simulink model "huzeyfe_ivot_462"  (R2018a)
settings: Solver=VariableStepAuto  StartTime=0.0  StopTime=10.0  RelTol=1e-3
libraries: powerlib x21, simulink x3, powerlib_meascontrol x1
settings Model: Creator=Gulten  LastModifiedBy=Gulten

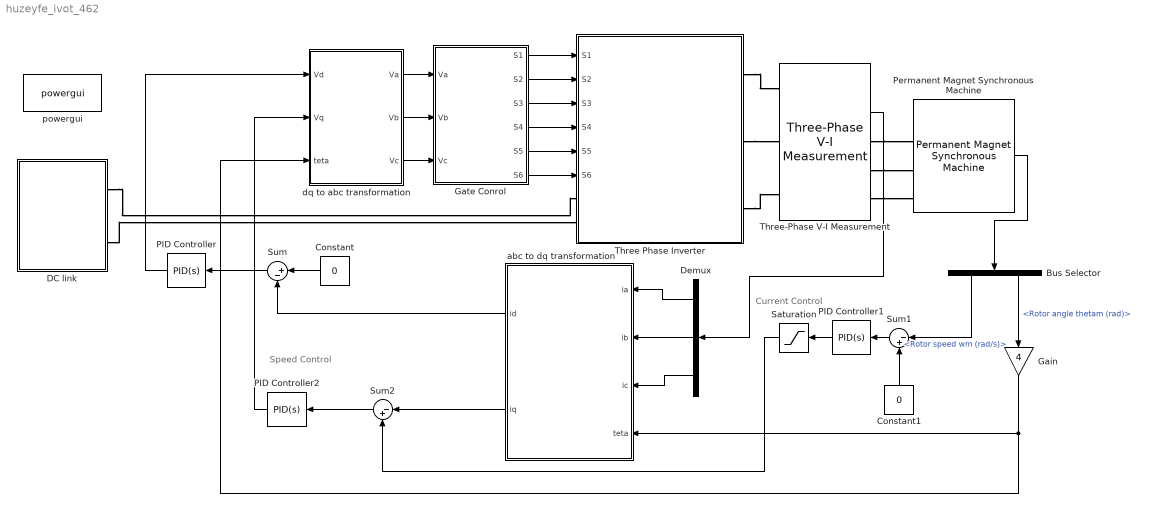
== system huzeyfe_ivot_462 ==
  note: Speed Control
  note: Current Control
  Bus Selector : BusSelector  OutputSignals=Rotor speed wm (rad/s),Rotor angle thetam (rad)
  Constant : Constant  Value=0
  Constant1 : Constant  Value=0
  DC link : Subsystem
  Demux : Demux  Outputs=3
  Gain : Gain  Gain=4
  Gate Conrol : Subsystem
  PID Controller : simulink/Continuous/PID Controller  Controller=PID  TimeDomain=Continuous-time  SampleTime=-1  IntegratorMethod=Forward Euler  FilterMethod=Forward Euler  Form=Parallel  UseFilter=on  ControllerParametersSource=internal  P=1  I=1  D=0  N=100  InitialConditionSource=internal  InitialConditionForIntegrator=0  InitialConditionForFilter=0  ExternalReset=none  LimitOutput=off  UpperSaturationLimit=inf  LowerSaturationLimit=-inf  LinearizeAsGain=on  AntiWindupMode=none  Kb=1  TrackingMode=off  Kt=1  PParamMin=[]  PParamMax=[]  IParamMin=[]  IParamMax=[]  DParamMin=[]  DParamMax=[]  NParamMin=[]  NParamMax=[]  KbParamMin=[]  KbParamMax=[]  KtParamMin=[]  KtParamMax=[]  POutMin=[]  POutMax=[]  IOutMin=[]  IOutMax=[]  DOutMin=[]  DOutMax=[]  NOutMin=[]  NOutMax=[]  KbOutMin=[]  KbOutMax=[]  KtOutMin=[]  KtOutMax=[]  IntegratorOutMin=[]  IntegratorOutMax=[]  FilterOutMin=[]  FilterOutMax=[]  SumOutMin=[]  SumOutMax=[]  SumI1OutMin=[]  SumI1OutMax=[]  SumI2OutMin=[]  SumI2OutMax=[]  SumI3OutMin=[]  SumI3OutMax=[]  SumDOutMin=[]  SumDOutMax=[]  SaturationOutMin=[]  SaturationOutMax=[]  IntegratorContinuousStateAttributes=''  IntegratorStateMustResolveToSignalObject=off  IntegratorRTWStateStorageClass=Auto  FilterContinuousStateAttributes=''  FilterStateMustResolveToSignalObject=off  FilterRTWStateStorageClass=Auto  DifferentiatorICPrevScaledInput=0  DifferentiatorOutMin=[]  DifferentiatorOutMax=[]  FilterDiffOutCoefMin=[]  FilterDiffOutCoefMax=[]  SumDenOutMin=[]  SumDenOutMax=[]  SumNumOutMin=[]  SumNumOutMax=[]  ReciprocalOutMin=[]  ReciprocalOutMax=[]  DivideOutMin=[]  DivideOutMax=[]  TunerSelectOption=Transfer Function Based (PID Tuner App)
  PID Controller1 : simulink/Continuous/PID Controller  Controller=PID  TimeDomain=Continuous-time  SampleTime=-1  IntegratorMethod=Forward Euler  FilterMethod=Forward Euler  Form=Parallel  UseFilter=on  ControllerParametersSource=internal  P=1  I=1  D=0  N=100  InitialConditionSource=internal  InitialConditionForIntegrator=0  InitialConditionForFilter=0  ExternalReset=none  LimitOutput=off  UpperSaturationLimit=inf  LowerSaturationLimit=-inf  LinearizeAsGain=on  AntiWindupMode=none  Kb=1  TrackingMode=off  Kt=1  PParamMin=[]  PParamMax=[]  IParamMin=[]  IParamMax=[]  DParamMin=[]  DParamMax=[]  NParamMin=[]  NParamMax=[]  KbParamMin=[]  KbParamMax=[]  KtParamMin=[]  KtParamMax=[]  POutMin=[]  POutMax=[]  IOutMin=[]  IOutMax=[]  DOutMin=[]  DOutMax=[]  NOutMin=[]  NOutMax=[]  KbOutMin=[]  KbOutMax=[]  KtOutMin=[]  KtOutMax=[]  IntegratorOutMin=[]  IntegratorOutMax=[]  FilterOutMin=[]  FilterOutMax=[]  SumOutMin=[]  SumOutMax=[]  SumI1OutMin=[]  SumI1OutMax=[]  SumI2OutMin=[]  SumI2OutMax=[]  SumI3OutMin=[]  SumI3OutMax=[]  SumDOutMin=[]  SumDOutMax=[]  SaturationOutMin=[]  SaturationOutMax=[]  IntegratorContinuousStateAttributes=''  IntegratorStateMustResolveToSignalObject=off  IntegratorRTWStateStorageClass=Auto  FilterContinuousStateAttributes=''  FilterStateMustResolveToSignalObject=off  FilterRTWStateStorageClass=Auto  DifferentiatorICPrevScaledInput=0  DifferentiatorOutMin=[]  DifferentiatorOutMax=[]  FilterDiffOutCoefMin=[]  FilterDiffOutCoefMax=[]  SumDenOutMin=[]  SumDenOutMax=[]  SumNumOutMin=[]  SumNumOutMax=[]  ReciprocalOutMin=[]  ReciprocalOutMax=[]  DivideOutMin=[]  DivideOutMax=[]  TunerSelectOption=Transfer Function Based (PID Tuner App)
  PID Controller2 : simulink/Continuous/PID Controller  Controller=PID  TimeDomain=Continuous-time  SampleTime=-1  IntegratorMethod=Forward Euler  FilterMethod=Forward Euler  Form=Parallel  UseFilter=on  ControllerParametersSource=internal  P=1  I=1  D=0  N=100  InitialConditionSource=internal  InitialConditionForIntegrator=0  InitialConditionForFilter=0  ExternalReset=none  LimitOutput=off  UpperSaturationLimit=inf  LowerSaturationLimit=-inf  LinearizeAsGain=on  AntiWindupMode=none  Kb=1  TrackingMode=off  Kt=1  PParamMin=[]  PParamMax=[]  IParamMin=[]  IParamMax=[]  DParamMin=[]  DParamMax=[]  NParamMin=[]  NParamMax=[]  KbParamMin=[]  KbParamMax=[]  KtParamMin=[]  KtParamMax=[]  POutMin=[]  POutMax=[]  IOutMin=[]  IOutMax=[]  DOutMin=[]  DOutMax=[]  NOutMin=[]  NOutMax=[]  KbOutMin=[]  KbOutMax=[]  KtOutMin=[]  KtOutMax=[]  IntegratorOutMin=[]  IntegratorOutMax=[]  FilterOutMin=[]  FilterOutMax=[]  SumOutMin=[]  SumOutMax=[]  SumI1OutMin=[]  SumI1OutMax=[]  SumI2OutMin=[]  SumI2OutMax=[]  SumI3OutMin=[]  SumI3OutMax=[]  SumDOutMin=[]  SumDOutMax=[]  SaturationOutMin=[]  SaturationOutMax=[]  IntegratorContinuousStateAttributes=''  IntegratorStateMustResolveToSignalObject=off  IntegratorRTWStateStorageClass=Auto  FilterContinuousStateAttributes=''  FilterStateMustResolveToSignalObject=off  FilterRTWStateStorageClass=Auto  DifferentiatorICPrevScaledInput=0  DifferentiatorOutMin=[]  DifferentiatorOutMax=[]  FilterDiffOutCoefMin=[]  FilterDiffOutCoefMax=[]  SumDenOutMin=[]  SumDenOutMax=[]  SumNumOutMin=[]  SumNumOutMax=[]  ReciprocalOutMin=[]  ReciprocalOutMax=[]  DivideOutMin=[]  DivideOutMax=[]  TunerSelectOption=Transfer Function Based (PID Tuner App)
  Permanent Magnet Synchronous Machine : powerlib/Machines/Permanent Magnet Synchronous Machine  NbPhases=3  FluxDistribution=Sinusoidal  RotorType=Round  MechanicalLoad=Torque Tm  PresetModel=No  ShowDetailedParameters=on  MeasurementBus=off  Resistance=50e-3  Inductance=8.5e-3  dqInductances=[500e-6,500e-6]  La=500e-6  MachineConstant=Flux linkage established by magnets (V.s)  Flux=0.2  VoltageCst=145.1039  TorqueCst=1.2  Flat=120  Mechanical=[10 0 4 0]  PolePairs=4  InitialConditions=[266,0, 0,0]  InitialConditions5ph=[266 0 0 0 0 0]  TsPowergui=0  TsBlock=-1  RefAngle=90 degrees behind phase A axis (modified Park)
      settings: SourceProductName=Simscape Power Systems
  Saturation : Saturate  UpperLimit=250  LowerLimit=-250
  Sum : Sum  Inputs=|+-
  Sum1 : Sum  Inputs=|-+
  Sum2 : Sum  Inputs=|-+
  Three Phase Inverter : Subsystem
  Three-Phase V-I Measurement : powerlib/Measurements/Three-Phase V-I Measurement  VoltageMeasurement=phase-to-phase  SetLabelV=off  LabelV=Vabc  Vpu=off  VpuLL=off  CurrentMeasurement=yes  SetLabelI=off  LabelI=Iabc  Ipu=off  Pbase=100e6  Vbase=500e3  OutputType=Complex  PhasorSimulation=off  PSBequivalent=0
  abc to dq transformation : Subsystem
  dq to abc transformation : Subsystem
  powergui : powerlib/powergui  Priority=1  SimulationMode=Discrete  SampleTime=5e-7  frequency=60  Iterations=50  frequencyindice=0  Pbase=100e6  ErrMax=1e-4  UnitsV=kV  UnitsW=MW  buscounter=0  FunctionMessages=off  echomessages=off  EnableUseOfTLC=off  CurrentSourceSwitches=off  DisableSnubberDevices=off  DisableRonSwitches=off  DisableVfSwitches=off  DisplayEquations=off  SolverType=Tustin/Backward Euler (TBE)  Interpol=off  ExternalGateDelay=off  methode=off  Ts=100  x0status=blocks  SPID=on  SwTol=0  HookPort=off  RestoreLinks=warning  ResistiveCurrentMeasurement=off  Frange=[0:2:500]  Ylog=off  Xlog=on  ShowGrid=off  save=off  variable=ZData  structure=0  ZoomFFT=off  StartTime=0.0  cycles=1  DisplayStyle=1  fundamental=60  FreqAxis=off  MaxFrequency=1000  frequencyindicesteady=1  RmsSteady=1  display=off
  wires:
  Gate Conrol/1(S1) -> Three Phase Inverter/1(S1)
  Gate Conrol/2(S2) -> Three Phase Inverter/2(S2)
  Gate Conrol/3(S3) -> Three Phase Inverter/3(S3)
  Gate Conrol/4(S4) -> Three Phase Inverter/4(S4)
  Gate Conrol/5(S5) -> Three Phase Inverter/5(S5)
  Gate Conrol/6(S6) -> Three Phase Inverter/6(S6)
  dq to abc transformation/1(Va) -> Gate Conrol/1(Va)
  dq to abc transformation/2(Vb) -> Gate Conrol/2(Vb)
  dq to abc transformation/3(Vc) -> Gate Conrol/3(Vc)
  Three-Phase V-I Measurement/2 -> Demux/1
  Demux/1 -> abc to dq transformation/1(ia)
  Demux/2 -> abc to dq transformation/2(ib)
  Demux/3 -> abc to dq transformation/3(ic)
  Permanent Magnet Synchronous Machine/1 -> Bus Selector/1
  Bus Selector/2 -> Gain/1  "<Rotor angle thetam (rad)>"
  abc to dq transformation/1(id) -> Sum/2
  Constant/1 -> Sum/1
  Sum/1 -> PID Controller/1
  PID Controller/1 -> dq to abc transformation/1(Vd)
  Gain/1 -> dq to abc transformation/3("teta "), abc to dq transformation/4(teta)
  Bus Selector/1 -> Sum1/1  "<Rotor speed wm (rad/s)>"
  Constant1/1 -> Sum1/2
  Sum1/1 -> PID Controller1/1
  abc to dq transformation/2(iq) -> Sum2/1
  Sum2/1 -> PID Controller2/1
  PID Controller2/1 -> dq to abc transformation/2(Vq)
  PID Controller1/1 -> Saturation/1
  Saturation/1 -> Sum2/2
  connections:
  DC link/RConn1 -- Three Phase Inverter/LConn1
  DC link/RConn2 -- Three Phase Inverter/LConn2
  Three Phase Inverter/RConn1 -- Three-Phase V-I Measurement/LConn1
  Three Phase Inverter/RConn2 -- Three-Phase V-I Measurement/LConn2
  Three Phase Inverter/RConn3 -- Three-Phase V-I Measurement/LConn3
  Three-Phase V-I Measurement/RConn1 -- Permanent Magnet Synchronous Machine/LConn1
  Three-Phase V-I Measurement/RConn2 -- Permanent Magnet Synchronous Machine/LConn2
  Three-Phase V-I Measurement/RConn3 -- Permanent Magnet Synchronous Machine/LConn3

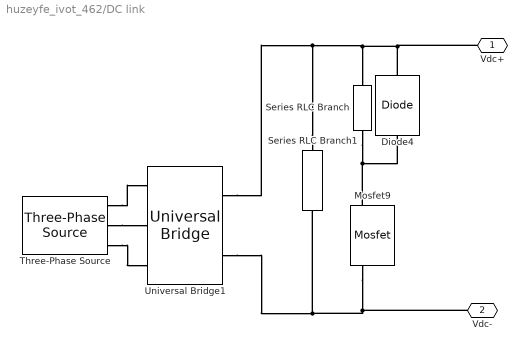
== system huzeyfe_ivot_462/DC link ==
  Diode4 : powerlib/Power Electronics/Diode  Ron=0.001  Lon=0  Vf=0  IC=0  UseSnubber=0  Rs=inf  Cs=inf  Measurements=off
  Mosfet9 : powerlib/Power Electronics/Mosfet  Ron=0.1  Lon=0  Rd=0.01  Vfd=0  IC=0  Rs=1e5  Cs=inf  Measurements=on
  Series RLC Branch : powerlib/Elements/Series RLC Branch  LConnTagsString=__new0  RConnTagsString=__new0  BranchType=R  Resistance=3  Inductance=1e-3  SetiL0=off  InitialCurrent=0  Capacitance=1e-6  Setx0=off  InitialVoltage=0  Measurements=None
  Series RLC Branch1 : powerlib/Elements/Series RLC Branch  LConnTagsString=__new0  RConnTagsString=__new0  BranchType=C  Resistance=1  Inductance=1e-3  SetiL0=off  InitialCurrent=0  Capacitance=1e-3  Setx0=off  InitialVoltage=0  Measurements=None
  Three-Phase Source : powerlib/Electrical Sources/Three-Phase Source  InternalConnection=Yg  VoltagePhases=off  Voltage=400  PhaseAngle=0  Voltage_phases=[25e3 25e3 25e3]/sqrt(3)  PhaseAngles_phases=[0 -120 +120]  Frequency=50  NonIdealSource=off  SpecifyImpedance=off  Resistance=0  Inductance=0  ShortCircuitLevel=100e6  BaseVoltage=25e3  XRratio=7  BusType=swing  Pref=10e3  Qref=0  Prefabc=[10e3, 10e3, 10e3]  Qrefabc=[0, 0, 0]  Qmin=-inf  Qmax=inf
  Universal Bridge1 : powerlib/Power Electronics/Universal Bridge  Arms=3  SnubberResistance=1e70  SnubberCapacitance=inf  Device=Diodes  Ron=1e-3  Lon=0  ForwardVoltages="[  0  0  ]"  ForwardVoltage=0  GTOparameters=[ 10e-6 , 20e-6 ]  IGBTparameters=[ 1e-6 , 2e-6 ]  Measurements=None  Measurements_2=None  converterType=Rectifier
  Vdc+ : PMIOPort  Side=Right
  Vdc- : PMIOPort  Port=2  Side=Right
  connections:
  Mosfet9/RConn1 -- Vdc-/RConn1 -- Universal Bridge1/RConn2 -- Series RLC Branch1/RConn1
  Series RLC Branch1/LConn1 -- Diode4/RConn1 -- Vdc+/RConn1 -- Series RLC Branch/LConn1 -- Universal Bridge1/RConn1
  Diode4/LConn1 -- Series RLC Branch/RConn1 -- Mosfet9/LConn1
  Three-Phase Source/RConn2 -- Universal Bridge1/LConn2
  Three-Phase Source/RConn3 -- Universal Bridge1/LConn3
  Three-Phase Source/RConn1 -- Universal Bridge1/LConn1

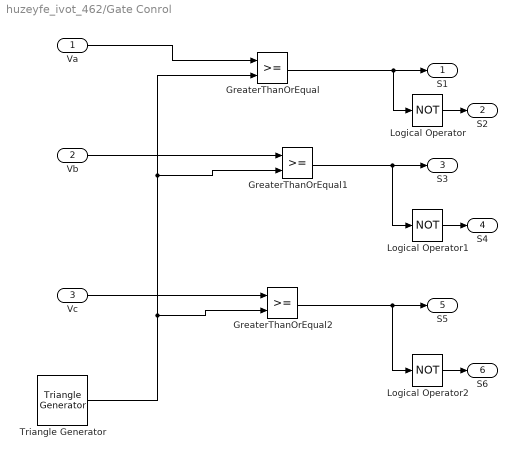
== system huzeyfe_ivot_462/Gate Conrol ==
  Va : Inport
  Vb : Inport  Port=2
  Vc : Inport  Port=3
  GreaterThanOrEqual : RelationalOperator  OutDataTypeStr=boolean  RndMeth=Simplest
  GreaterThanOrEqual1 : RelationalOperator  OutDataTypeStr=boolean  RndMeth=Simplest
  GreaterThanOrEqual2 : RelationalOperator  OutDataTypeStr=boolean  RndMeth=Simplest
  Logical Operator : Logic  Operator=NOT  AllPortsSameDT=off  OutDataTypeStr=boolean
  Logical Operator1 : Logic  Operator=NOT  AllPortsSameDT=off  OutDataTypeStr=boolean
  Logical Operator2 : Logic  Operator=NOT  AllPortsSameDT=off  OutDataTypeStr=boolean
  Triangle Generator : powerlib_meascontrol/Pulse & Signal Generators/Triangle Generator  Freq=5330  Phase=90  Ts=0
  S1 : Outport
  S2 : Outport  Port=2
  S3 : Outport  Port=3
  S4 : Outport  Port=4
  S5 : Outport  Port=5
  S6 : Outport  Port=6
  wires:
  Vc/1 -> GreaterThanOrEqual2/1
  Logical Operator2/1 -> S6/1
  Logical Operator1/1 -> S4/1
  Logical Operator/1 -> S2/1
  GreaterThanOrEqual1/1 -> S3/1, Logical Operator1/1
  GreaterThanOrEqual2/1 -> S5/1, Logical Operator2/1
  Va/1 -> GreaterThanOrEqual/1
  GreaterThanOrEqual/1 -> S1/1, Logical Operator/1
  Triangle Generator/1 -> GreaterThanOrEqual2/2, GreaterThanOrEqual/2, GreaterThanOrEqual1/2
  Vb/1 -> GreaterThanOrEqual1/1

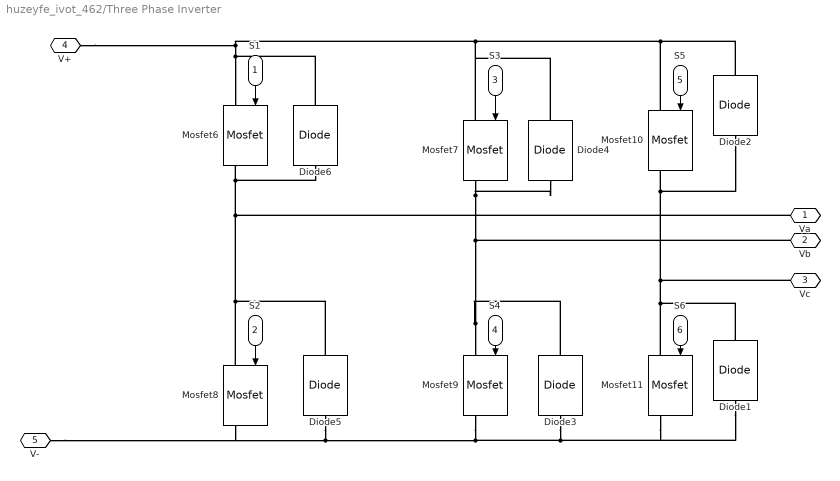
== system huzeyfe_ivot_462/Three Phase Inverter ==
  S1 : Inport
  S2 : Inport  Port=2
  S3 : Inport  Port=3
  S4 : Inport  Port=4
  S5 : Inport  Port=5
  S6 : Inport  Port=6
  Diode{1..6} (6 alike) : powerlib/Power Electronics/Diode  Ron=0.001  Lon=0  Vf=0  IC=0  UseSnubber=0  Rs=inf  Cs=inf  Measurements=off
  Mosfet{6..11} (6 alike) : powerlib/Power Electronics/Mosfet  Ron=0.1  Lon=0  Rd=0.01  Vfd=0  IC=0  Rs=1e5  Cs=inf  Measurements=on
  Va : PMIOPort  Side=Right
  Vb : PMIOPort  Port=2  Side=Right
  Vc : PMIOPort  Port=3  Side=Right
  V+ : PMIOPort  Port=4  Side=Left
  V- : PMIOPort  Port=5  Side=Left
  wires:
  S1/1 -> Mosfet6/1
  S2/1 -> Mosfet8/1
  S3/1 -> Mosfet7/1
  S4/1 -> Mosfet9/1
  S5/1 -> Mosfet10/1
  S6/1 -> Mosfet11/1
  connections:
  Mosfet9/RConn1 -- Diode1/LConn1 -- Mosfet11/RConn1 -- Diode3/LConn1 -- V-/RConn1 -- Mosfet8/RConn1 -- Diode5/LConn1
  Mosfet7/RConn1 -- Vb/RConn1 -- Diode3/RConn1 -- Mosfet9/LConn1 -- Diode4/LConn1
  Mosfet10/LConn1 -- Diode2/RConn1 -- Diode4/RConn1 -- Mosfet7/LConn1 -- V+/RConn1 -- Diode6/RConn1 -- Mosfet6/LConn1
  Mosfet8/LConn1 -- Diode5/RConn1 -- Va/RConn1 -- Diode6/LConn1 -- Mosfet6/RConn1
  Mosfet11/LConn1 -- Diode1/RConn1 -- Vc/RConn1 -- Diode2/LConn1 -- Mosfet10/RConn1

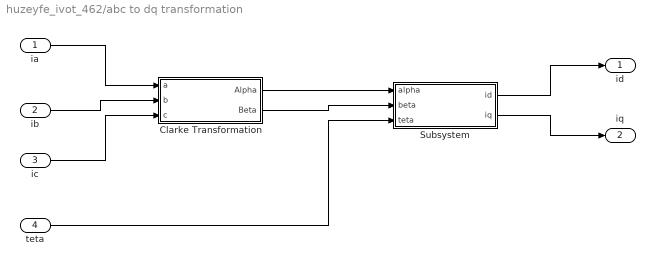
== system huzeyfe_ivot_462/abc to dq transformation ==
  ia : Inport
  ib : Inport  Port=2
  ic : Inport  Port=3
  teta : Inport  Port=4
  Clarke Transformation : Subsystem
  Subsystem : Subsystem
  id : Outport
  iq : Outport  Port=2
  wires:
  ia/1 -> Clarke Transformation/1(a)
  ib/1 -> Clarke Transformation/2(b)
  ic/1 -> Clarke Transformation/3(c)
  teta/1 -> Subsystem/3(teta)
  Clarke Transformation/2(Beta) -> Subsystem/2(beta)
  Clarke Transformation/1(Alpha) -> Subsystem/1(alpha)
  Subsystem/1(id) -> id/1
  Subsystem/2(iq) -> iq/1

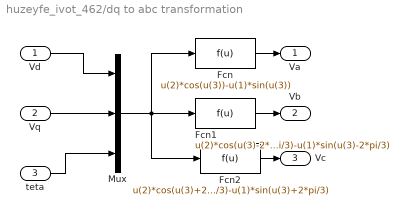
== system huzeyfe_ivot_462/dq to abc transformation ==
  Vd : Inport
  Vq : Inport  Port=2
  "teta " : Inport  Port=3
  Fcn : Fcn  Expr=u(2)*cos(u(3))-u(1)*sin(u(3))
  Fcn1 : Fcn  Expr=u(2)*cos(u(3)-2*pi/3)-u(1)*sin(u(3)-2*pi/3)
  Fcn2 : Fcn  Expr=u(2)*cos(u(3)+2*pi/3)-u(1)*sin(u(3)+2*pi/3)
  Mux : Mux  Inputs=3
  Va : Outport
  Vb : Outport  Port=2
  Vc : Outport  Port=3
  wires:
  Mux/1 -> Fcn/1, Fcn2/1, Fcn1/1
  Fcn1/1 -> Vb/1
  Vd/1 -> Mux/1
  Fcn/1 -> Va/1
  Vq/1 -> Mux/2
  "teta "/1 -> Mux/3
  Fcn2/1 -> Vc/1

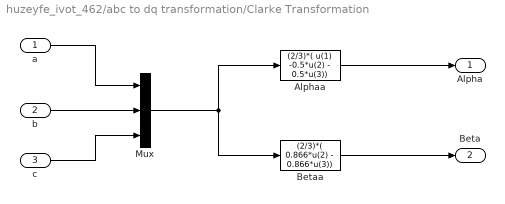
== system huzeyfe_ivot_462/abc to dq transformation/Clarke Transformation ==
  a : Inport
  b : Inport  Port=2
  c : Inport  Port=3
  Alphaa : Fcn  Expr=(2/3)*( u(1) -0.5*u(2) - 0.5*u(3))
  Betaa : Fcn  Expr=(2/3)*( 0.866*u(2) - 0.866*u(3))
  Mux : Mux  Inputs=3
  Alpha : Outport
  Beta : Outport  Port=2
  wires:
  a/1 -> Mux/1
  b/1 -> Mux/2
  c/1 -> Mux/3
  Betaa/1 -> Beta/1
  Alphaa/1 -> Alpha/1
  Mux/1 -> Alphaa/1, Betaa/1

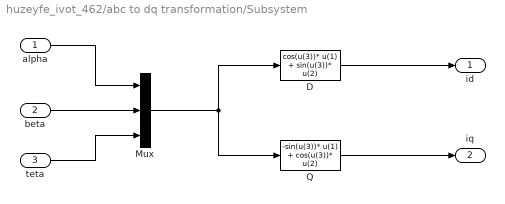
== system huzeyfe_ivot_462/abc to dq transformation/Subsystem ==
  alpha : Inport
  beta : Inport  Port=2
  teta : Inport  Port=3
  D : Fcn  Expr=cos(u(3))* u(1) + sin(u(3))* u(2)
  Mux : Mux  Inputs=3
  Q : Fcn  Expr=-sin(u(3))* u(1) + cos(u(3))* u(2)
  id : Outport
  iq : Outport  Port=2
  wires:
  Mux/1 -> D/1, Q/1
  teta/1 -> Mux/3
  beta/1 -> Mux/2
  alpha/1 -> Mux/1
  D/1 -> id/1
  Q/1 -> iq/1
